simulink model "stage1_ddc"  (R2012b)
settings: Solver=FixedStepDiscrete  SolverMode=SingleTasking  StartTime=0.0  StopTime=T  RelTol=1e-3
undefined symbols (not defined in the file): cb0, cb1, cb2, cb3, cb4, cb5, cb6, cb7, dphi, Dphi, phi0
libraries: xbsIndex_r4 x332, unit_testing x23, filters x8, r2daq_blocks x5, synths x1, xps_library x1
(part 1 of 10)
settings Model: Creator=ayoung  LastModifiedBy=ayoung

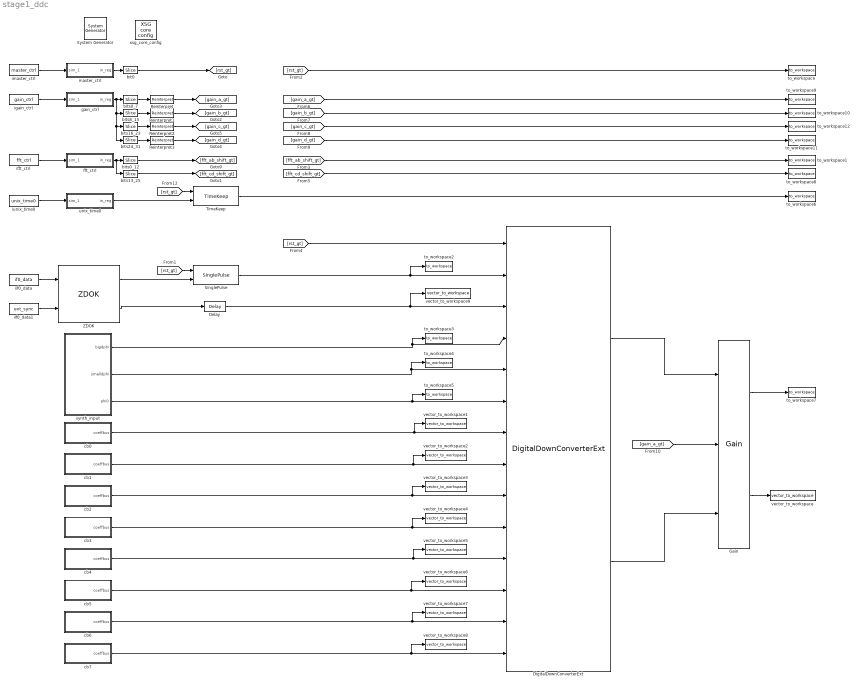
== system stage1_ddc ==
  " System Generator" : xbsIndex_r4/ System Generator  Tag=genX  xilinxfamily=Kintex7  part=xc7k325t  speed=-3  package=fbg676  synthesis_tool=XST  clock_wrapper=Clock Enables  directory=./netlist  proj_type=Project Navigator  Synth_file=XST Defaults  Impl_file=ISE Defaults  testbench=off  simulink_period=1  sysclk_period=10  dcm_input_clock_period=10  incr_netlist=off  trim_vbits=Everywhere in SubSystem  dbl_ovrd=According to Block Masks  core_generation=According to Block Masks  run_coregen=off  deprecated_control=off  eval_field=0  block_type=sysgen
  Delay : xbsIndex_r4/Delay  rst=off  infoeditControl=Selection of Reset will increase slice count due to use of real FFs and instead of SRLs  en=off  latency=1  dbl_ovrd=off  reg_retiming=off  block_type=delay
  DigitalDownConverterExt : r2daq_blocks/DigitalDownConverterExt
      link override bus_mul_cosine/a_debus: outputNum=1
      link override bus_mul_cosine/b_debus: outputNum=1
      link override bus_mul_sine/a_debus: outputNum=1
      link override bus_mul_sine/b_debus: outputNum=1
      link override ifir/bus_del1/din_expand: outputNum=1
      link override ifir/bus_del2/din_expand: outputNum=1
      link override ifir/bus_del3/din_expand: outputNum=1
      link override ifir/bus_del4/din_expand: outputNum=1
      link override ifir/bus_del5/din_expand: outputNum=1
      link override ifir/bus_del6/din_expand: outputNum=1
      link override ifir/bus_del7/din_expand: outputNum=1
      link override ifir/bus_mul0/a_debus: outputNum=1
      link override ifir/bus_mul0/b_debus: outputNum=1
      link override ifir/bus_mul1/a_debus: outputNum=1
      link override ifir/bus_mul1/b_debus: outputNum=1
      link override ifir/bus_mul2/a_debus: outputNum=1
      link override ifir/bus_mul2/b_debus: outputNum=1
      link override ifir/bus_mul3/a_debus: outputNum=1
      link override ifir/bus_mul3/b_debus: outputNum=1
      link override ifir/bus_mul4/a_debus: outputNum=1
      link override ifir/bus_mul4/b_debus: outputNum=1
      link override ifir/bus_mul5/a_debus: outputNum=1
      link override ifir/bus_mul5/b_debus: outputNum=1
      link override ifir/bus_mul6/a_debus: outputNum=1
      link override ifir/bus_mul6/b_debus: outputNum=1
      link override ifir/bus_mul7/a_debus: outputNum=1
      link override ifir/bus_mul7/b_debus: outputNum=1
      link override qfir/bus_del1/din_expand: outputNum=1
      link override qfir/bus_del2/din_expand: outputNum=1
      link override qfir/bus_del3/din_expand: outputNum=1
      link override qfir/bus_del4/din_expand: outputNum=1
      link override qfir/bus_del5/din_expand: outputNum=1
      link override qfir/bus_del6/din_expand: outputNum=1
      link override qfir/bus_del7/din_expand: outputNum=1
      link override qfir/bus_mul0/a_debus: outputNum=1
      link override qfir/bus_mul0/b_debus: outputNum=1
      link override qfir/bus_mul1/a_debus: outputNum=1
      link override qfir/bus_mul1/b_debus: outputNum=1
      link override qfir/bus_mul2/a_debus: outputNum=1
      link override qfir/bus_mul2/b_debus: outputNum=1
      link override qfir/bus_mul3/a_debus: outputNum=1
      link override qfir/bus_mul3/b_debus: outputNum=1
      link override qfir/bus_mul4/a_debus: outputNum=1
      link override qfir/bus_mul4/b_debus: outputNum=1
      link override qfir/bus_mul5/a_debus: outputNum=1
      link override qfir/bus_mul5/b_debus: outputNum=1
      link override qfir/bus_mul6/a_debus: outputNum=1
      link override qfir/bus_mul6/b_debus: outputNum=1
      link override qfir/bus_mul7/a_debus: outputNum=1
      link override qfir/bus_mul7/b_debus: outputNum=1
  Gain : r2daq_blocks/Gain
  Reinterpret{,1..3} (4 alike) : xbsIndex_r4/Reinterpret  force_arith_type=on  arith_type="Signed  (2's comp)"  force_bin_pt=on  bin_pt=4  block_type=reinterpret
  SinglePulse : r2daq_blocks/SinglePulse
  TimeKeep : r2daq_blocks/TimeKeep
  ZDOK : r2daq_blocks/ZDOK  zdok_slot=ZDOK 1  freq_nyq=1600
      link override asiaa_adc5g/a0: Port=1
      link override asiaa_adc5g/a1: Port=2
      link override asiaa_adc5g/a10: Port=11
      link override asiaa_adc5g/a11: Port=12
      link override asiaa_adc5g/a12: Port=13
      link override asiaa_adc5g/a13: Port=14
      link override asiaa_adc5g/a14: Port=15
      link override asiaa_adc5g/a15: Port=16
      link override asiaa_adc5g/a2: Port=3
      link override asiaa_adc5g/a3: Port=4
      link override asiaa_adc5g/a4: Port=5
      link override asiaa_adc5g/a5: Port=6
      link override asiaa_adc5g/a6: Port=7
      link override asiaa_adc5g/a7: Port=8
      link override asiaa_adc5g/a8: Port=9
      link override asiaa_adc5g/a9: Port=10
      link override asiaa_adc5g/bias_a: Bias=128
      link override asiaa_adc5g/delay_a0: DelayLength=2
      link override asiaa_adc5g/delay_a1: DelayLength=1
      link override asiaa_adc5g/delay_a10: DelayLength=1
      link override asiaa_adc5g/delay_a11: DelayLength=1
      link override asiaa_adc5g/delay_a12: DelayLength=1
      link override asiaa_adc5g/delay_a13: DelayLength=1
      link override asiaa_adc5g/delay_a14: DelayLength=1
      link override asiaa_adc5g/delay_a15: DelayLength=1
      link override asiaa_adc5g/delay_a2: DelayLength=1
      link override asiaa_adc5g/delay_a3: DelayLength=1
      link override asiaa_adc5g/delay_a4: DelayLength=1
      link override asiaa_adc5g/delay_a5: DelayLength=1
      link override asiaa_adc5g/delay_a6: DelayLength=1
      link override asiaa_adc5g/delay_a7: DelayLength=1
      link override asiaa_adc5g/delay_a8: DelayLength=1
      link override asiaa_adc5g/delay_a9: DelayLength=1
      link override asiaa_adc5g/downsample_a0: N=16  phase=0  RateOptions=Allow multirate processing  ic=0
      link override asiaa_adc5g/downsample_a1: N=16  phase=1  RateOptions=Allow multirate processing  ic=0
      link override asiaa_adc5g/downsample_a10: N=16  phase=10  RateOptions=Allow multirate processing  ic=0
      link override asiaa_adc5g/downsample_a11: N=16  phase=11  RateOptions=Allow multirate processing  ic=0
      link override asiaa_adc5g/downsample_a12: N=16  phase=12  RateOptions=Allow multirate processing  ic=0
      link override asiaa_adc5g/downsample_a13: N=16  phase=13  RateOptions=Allow multirate processing  ic=0
      link override asiaa_adc5g/downsample_a14: N=16  phase=14  RateOptions=Allow multirate processing  ic=0
      link override asiaa_adc5g/downsample_a15: N=16  phase=15  RateOptions=Allow multirate processing  ic=0
      link override asiaa_adc5g/downsample_a2: N=16  phase=2  RateOptions=Allow multirate processing  ic=0
      link override asiaa_adc5g/downsample_a3: N=16  phase=3  RateOptions=Allow multirate processing  ic=0
      link override asiaa_adc5g/downsample_a4: N=16  phase=4  RateOptions=Allow multirate processing  ic=0
      link override asiaa_adc5g/downsample_a5: N=16  phase=5  RateOptions=Allow multirate processing  ic=0
      link override asiaa_adc5g/downsample_a6: N=16  phase=6  RateOptions=Allow multirate processing  ic=0
      link override asiaa_adc5g/downsample_a7: N=16  phase=7  RateOptions=Allow multirate processing  ic=0
      link override asiaa_adc5g/downsample_a8: N=16  phase=8  RateOptions=Allow multirate processing  ic=0
      link override asiaa_adc5g/downsample_a9: N=16  phase=9  RateOptions=Allow multirate processing  ic=0
      link override asiaa_adc5g/gain_a: Gain=128
      link override asiaa_adc5g/sim_a: Port=1
      link override asiaa_adc5g/sim_sync: Port=2
      link override asiaa_adc5g/simulink_need_slupdate_PID_Controller_with_Approximate_Derivative_sync: arith_type=Boolean
      link override asiaa_adc5g/simulink_need_slupdate_PID_Controller_with_Approximate_Derivative_user_data_i0: arith_type=Unsigned  n_bits=8  bin_pt=0  quantization=Truncate  overflow=Wrap
      link override asiaa_adc5g/simulink_need_slupdate_PID_Controller_with_Approximate_Derivative_user_data_i1: arith_type=Unsigned  n_bits=8  bin_pt=0  quantization=Truncate  overflow=Wrap
      link override asiaa_adc5g/simulink_need_slupdate_PID_Controller_with_Approximate_Derivative_user_data_i2: arith_type=Unsigned  n_bits=8  bin_pt=0  quantization=Truncate  overflow=Wrap
      link override asiaa_adc5g/simulink_need_slupdate_PID_Controller_with_Approximate_Derivative_user_data_i3: arith_type=Unsigned  n_bits=8  bin_pt=0  quantization=Truncate  overflow=Wrap
      link override asiaa_adc5g/simulink_need_slupdate_PID_Controller_with_Approximate_Derivative_user_data_i4: arith_type=Unsigned  n_bits=8  bin_pt=0  quantization=Truncate  overflow=Wrap
      link override asiaa_adc5g/simulink_need_slupdate_PID_Controller_with_Approximate_Derivative_user_data_i5: arith_type=Unsigned  n_bits=8  bin_pt=0  quantization=Truncate  overflow=Wrap
      link override asiaa_adc5g/simulink_need_slupdate_PID_Controller_with_Approximate_Derivative_user_data_i6: arith_type=Unsigned  n_bits=8  bin_pt=0  quantization=Truncate  overflow=Wrap
      link override asiaa_adc5g/simulink_need_slupdate_PID_Controller_with_Approximate_Derivative_user_data_i7: arith_type=Unsigned  n_bits=8  bin_pt=0  quantization=Truncate  overflow=Wrap
      link override asiaa_adc5g/simulink_need_slupdate_PID_Controller_with_Approximate_Derivative_user_data_q0: arith_type=Unsigned  n_bits=8  bin_pt=0  quantization=Truncate  overflow=Wrap
      link override asiaa_adc5g/simulink_need_slupdate_PID_Controller_with_Approximate_Derivative_user_data_q1: arith_type=Unsigned  n_bits=8  bin_pt=0  quantization=Truncate  overflow=Wrap
      link override asiaa_adc5g/simulink_need_slupdate_PID_Controller_with_Approximate_Derivative_user_data_q2: arith_type=Unsigned  n_bits=8  bin_pt=0  quantization=Truncate  overflow=Wrap
      link override asiaa_adc5g/simulink_need_slupdate_PID_Controller_with_Approximate_Derivative_user_data_q3: arith_type=Unsigned  n_bits=8  bin_pt=0  quantization=Truncate  overflow=Wrap
      link override asiaa_adc5g/simulink_need_slupdate_PID_Controller_with_Approximate_Derivative_user_data_q4: arith_type=Unsigned  n_bits=8  bin_pt=0  quantization=Truncate  overflow=Wrap
      link override asiaa_adc5g/simulink_need_slupdate_PID_Controller_with_Approximate_Derivative_user_data_q5: arith_type=Unsigned  n_bits=8  bin_pt=0  quantization=Truncate  overflow=Wrap
      link override asiaa_adc5g/simulink_need_slupdate_PID_Controller_with_Approximate_Derivative_user_data_q6: arith_type=Unsigned  n_bits=8  bin_pt=0  quantization=Truncate  overflow=Wrap
      link override asiaa_adc5g/simulink_need_slupdate_PID_Controller_with_Approximate_Derivative_user_data_q7: arith_type=Unsigned  n_bits=8  bin_pt=0  quantization=Truncate  overflow=Wrap
      link override asiaa_adc5g/sync_out: Port=17
  bit0 : xbsIndex_r4/Slice  nbits=1  boolean_output=on  mode=Lower Bit Location + Width  bit1=0  base1=LSB of Input  bit0=0  base0=LSB of Input  dbl_ovrd=off  block_type=slice
  bits0_12 : xbsIndex_r4/Slice  nbits=13  boolean_output=off  mode=Lower Bit Location + Width  bit1=0  base1=LSB of Input  bit0=0  base0=LSB of Input  dbl_ovrd=off  block_type=slice
  bits0_7 : xbsIndex_r4/Slice  nbits=8  boolean_output=off  mode=Lower Bit Location + Width  bit1=0  base1=LSB of Input  bit0=0  base0=LSB of Input  dbl_ovrd=off  block_type=slice
  bits13_25 : xbsIndex_r4/Slice  nbits=13  boolean_output=off  mode=Lower Bit Location + Width  bit1=0  base1=LSB of Input  bit0=13  base0=LSB of Input  dbl_ovrd=off  block_type=slice
  bits16_23 : xbsIndex_r4/Slice  nbits=8  boolean_output=off  mode=Lower Bit Location + Width  bit1=0  base1=LSB of Input  bit0=8  base0=LSB of Input  dbl_ovrd=off  block_type=slice
  bits24_31 : xbsIndex_r4/Slice  nbits=8  boolean_output=off  mode=Lower Bit Location + Width  bit1=0  base1=LSB of Input  bit0=8  base0=LSB of Input  dbl_ovrd=off  block_type=slice
  bits8_15 : xbsIndex_r4/Slice  nbits=8  boolean_output=off  mode=Lower Bit Location + Width  bit1=0  base1=LSB of Input  bit0=8  base0=LSB of Input  dbl_ovrd=off  block_type=slice
  cb0 : Subsystem  AncestorBlock=filters/coeff_16x8bit_bus  mask(coeff_16x8bit_bus){io_delay=3, sim_in=on, coeff=cb0}
      mask prompts: io_delay "I/O delay for registers"; sim_in "Provide sim input?"; coeff "Coefficients (4 x uint32)"
      mask help:
      | Provides 16x8bit coefficients on a single bus.
      |
      | The coefficients are set in 4x32bit software registers.
      |
      | The I/O delay of the internal registers can be set, as well as an optional simulation input to each.
      mask init:
      | %for ii=0:3
      | %    swr = [gcb sprintf('/g%d',ii)];
      | %    set_param(swr,'sim_port',sim_in);
      | %    set_param(swr,'io_delay',num2str(io_delay));
      | %end
      | coeff_16x8bit_bus_init(gcb,...
      |     'io_delay',io_delay,...
      |     'sim_in',sim_in,...
      |     'coeff',coeff);
      mask Callback sim_in:
      | if strcmpi(get_param(gcb,'sim_in'),'off')
      |     set_param(gcb,'MaskEnables',{'on';'on';'off'});
      | else
      |     set_param(gcb,'MaskEnables',{'on';'on';'on'});
      | end
  cb1 : Subsystem  AncestorBlock=filters/coeff_16x8bit_bus  mask(coeff_16x8bit_bus){io_delay=3, sim_in=on, coeff=cb1}
      mask prompts: io_delay "I/O delay for registers"; sim_in "Provide sim input?"; coeff "Coefficients (4 x uint32)"
      mask help:
      | Provides 16x8bit coefficients on a single bus.
      |
      | The coefficients are set in 4x32bit software registers.
      |
      | The I/O delay of the internal registers can be set, as well as an optional simulation input to each.
      mask init: same as stage1_ddc/cb0
      mask Callback sim_in:
      | if strcmpi(get_param(gcb,'sim_in'),'off')
      |     set_param(gcb,'MaskEnables',{'on';'on';'off'});
      | else
      |     set_param(gcb,'MaskEnables',{'on';'on';'on'});
      | end
  cb2 : Subsystem  AncestorBlock=filters/coeff_16x8bit_bus  mask(coeff_16x8bit_bus){io_delay=3, sim_in=on, coeff=cb2}
      mask prompts: io_delay "I/O delay for registers"; sim_in "Provide sim input?"; coeff "Coefficients (4 x uint32)"
      mask help:
      | Provides 16x8bit coefficients on a single bus.
      |
      | The coefficients are set in 4x32bit software registers.
      |
      | The I/O delay of the internal registers can be set, as well as an optional simulation input to each.
      mask init: same as stage1_ddc/cb0
      mask Callback sim_in:
      | if strcmpi(get_param(gcb,'sim_in'),'off')
      |     set_param(gcb,'MaskEnables',{'on';'on';'off'});
      | else
      |     set_param(gcb,'MaskEnables',{'on';'on';'on'});
      | end
  cb3 : Subsystem  AncestorBlock=filters/coeff_16x8bit_bus  mask(coeff_16x8bit_bus){io_delay=3, sim_in=on, coeff=cb3}
      mask prompts: io_delay "I/O delay for registers"; sim_in "Provide sim input?"; coeff "Coefficients (4 x uint32)"
      mask help:
      | Provides 16x8bit coefficients on a single bus.
      |
      | The coefficients are set in 4x32bit software registers.
      |
      | The I/O delay of the internal registers can be set, as well as an optional simulation input to each.
      mask init: same as stage1_ddc/cb0
      mask Callback sim_in:
      | if strcmpi(get_param(gcb,'sim_in'),'off')
      |     set_param(gcb,'MaskEnables',{'on';'on';'off'});
      | else
      |     set_param(gcb,'MaskEnables',{'on';'on';'on'});
      | end
  cb4 : Subsystem  AncestorBlock=filters/coeff_16x8bit_bus  mask(coeff_16x8bit_bus){io_delay=3, sim_in=on, coeff=cb4}
      mask prompts: io_delay "I/O delay for registers"; sim_in "Provide sim input?"; coeff "Coefficients (4 x uint32)"
      mask help:
      | Provides 16x8bit coefficients on a single bus.
      |
      | The coefficients are set in 4x32bit software registers.
      |
      | The I/O delay of the internal registers can be set, as well as an optional simulation input to each.
      mask init: same as stage1_ddc/cb0
      mask Callback sim_in:
      | if strcmpi(get_param(gcb,'sim_in'),'off')
      |     set_param(gcb,'MaskEnables',{'on';'on';'off'});
      | else
      |     set_param(gcb,'MaskEnables',{'on';'on';'on'});
      | end
  cb5 : Subsystem  AncestorBlock=filters/coeff_16x8bit_bus  mask(coeff_16x8bit_bus){io_delay=3, sim_in=on, coeff=cb5}
      mask prompts: io_delay "I/O delay for registers"; sim_in "Provide sim input?"; coeff "Coefficients (4 x uint32)"
      mask help:
      | Provides 16x8bit coefficients on a single bus.
      |
      | The coefficients are set in 4x32bit software registers.
      |
      | The I/O delay of the internal registers can be set, as well as an optional simulation input to each.
      mask init: same as stage1_ddc/cb0
      mask Callback sim_in:
      | if strcmpi(get_param(gcb,'sim_in'),'off')
      |     set_param(gcb,'MaskEnables',{'on';'on';'off'});
      | else
      |     set_param(gcb,'MaskEnables',{'on';'on';'on'});
      | end
  cb6 : Subsystem  AncestorBlock=filters/coeff_16x8bit_bus  mask(coeff_16x8bit_bus){io_delay=3, sim_in=on, coeff=cb6}
      mask prompts: io_delay "I/O delay for registers"; sim_in "Provide sim input?"; coeff "Coefficients (4 x uint32)"
      mask help:
      | Provides 16x8bit coefficients on a single bus.
      |
      | The coefficients are set in 4x32bit software registers.
      |
      | The I/O delay of the internal registers can be set, as well as an optional simulation input to each.
      mask init: same as stage1_ddc/cb0
      mask Callback sim_in:
      | if strcmpi(get_param(gcb,'sim_in'),'off')
      |     set_param(gcb,'MaskEnables',{'on';'on';'off'});
      | else
      |     set_param(gcb,'MaskEnables',{'on';'on';'on'});
      | end
  cb7 : Subsystem  AncestorBlock=filters/coeff_16x8bit_bus  mask(coeff_16x8bit_bus){io_delay=3, sim_in=on, coeff=cb7}
      mask prompts: io_delay "I/O delay for registers"; sim_in "Provide sim input?"; coeff "Coefficients (4 x uint32)"
      mask help:
      | Provides 16x8bit coefficients on a single bus.
      |
      | The coefficients are set in 4x32bit software registers.
      |
      | The I/O delay of the internal registers can be set, as well as an optional simulation input to each.
      mask init: same as stage1_ddc/cb0
      mask Callback sim_in:
      | if strcmpi(get_param(gcb,'sim_in'),'off')
      |     set_param(gcb,'MaskEnables',{'on';'on';'off'});
      | else
      |     set_param(gcb,'MaskEnables',{'on';'on';'on'});
      | end
  fft_ctrl : Subsystem  Tag=xps:sw_reg  AncestorBlock=xps_library/software_register  mask(swreg){mode=one value, io_dir=From Processor, io_delay=0, sample_period=1, names=reg, bitwidths=32, arith_types=0, bin_pts=0, sim_port=on, show_format=off}
      mask prompts: io_dir "I/O direction"; io_delay "I/O delay"; sample_period "Sample period"; names "Name:"; bitwidths "Bitwidth:"; arith_types "Type (ufix=0, fix=1, bool=2):"; bin_pts "Binary pt:"; sim_port "Provide sim input/output?"; show_format "Print format string?"
      mask init:
      | swreg_init(gcb)
      settings: AttributesFormatString=1input
      mask TypeOptions mode: one value | fields of equal size | fields of arbitrary size
      mask Callback mode: swreg_cb(gcb);
      mask TypeOptions io_dir: To Processor | From Processor
      mask Callback io_dir:
      | mask_enables = get_param(gcb, 'MaskEnables');
      | mask_names = get_param(gcb, 'MaskNames');
      | if strcmp(get_param(gcb, 'io_dir'), 'To Processor'),
      |     mask_enables{ismember(mask_names, 'sample_period')} = 'off';
      | else
      |     mask_enables{ismember(mask_names, 'sample_period')} = 'on';
      | end
      | set_param(gcb, 'MaskEnables', mask_enables);
      mask Callback bitwidths:
      | swreg_maskcheck(gcb);
      | % blk = gcb;
      | % mode = get_param(blk, 'mode');
      | % current_widths = eval(get_param(blk, 'bitwidths'));
      | % if (strcmp(mode, 'one value') || strcmp(mode, 'fields of equal size')) && (length(current_widths) > 1),
      | %     error('Only one width may be specified for this mode.');
      | % elseif strcmp(mode, 'fields of arbitrary size')
      | %     current_names = textscan(strtrim(strrep(strrep(get_param(blk, 'names'), ']', ''), '[', '')), '%s');
      | %     current_names = current_names{1};
      | %     numios = length(current_names);
      | %     if length(current_widths) ~= numios,
      | %         error('%d field names specified, but %d widths?', numios, length(current_widths));
      | %     end
      | % end
      | % total_width = 0;
      | % for ctr = 1 : length(current_widths),
      | %     total_width = total_width + current_widths(ctr);
      | % end
      | % if total_width > 32,
      | %     error('Total width must be 32 or less, set to %d.', total_width);
      | % end
      mask Callback arith_types:
      | [numios, ~, ~, ~, current_types] = swreg_maskcheck(gcb);
      | % blk = gcb;
      | % mode = get_param(blk, 'mode');
      | % current_types = eval(get_param(blk, 'arith_types'));
      | % numios = length(current_types);
      | % if (strcmp(mode, 'one value') || strcmp(mode, 'fields of equal size')) && (length(current_types) > 1),
      | %     error('Only one type may be specified for this mode.');
      | % elseif strcmp(mode, 'fields of arbitrary size')
      | %     current_names = textscan(strtrim(strrep(strrep(get_param(blk, 'names'), ']', ''), '[', '')), '%s');
      | %     current_names = current_names{1};
      | %     numios = length(current_names);
      | %     if length(current_types) ~= numios,
      | %         error('%d field names specified, but %d types?', numios, length(current_types));
      | %     end
      | % end
      | problem = 0;
      | for ctr = 1 : numios,
      |     t = current_types(ctr);
      |     if (t < 0) || (t > 2),
      |         problem = t;
      |         ctr = numios + 1;
      |     end
      | end
      | if problem ~= 0,
      |     error('Type cannot be %i, must be 0, 1 or 2.', problem);
      | end
      mask Callback bin_pts:
      | swreg_maskcheck(gcb);
      | % blk = gcb;
      | % mode = get_param(blk, 'mode');
      | % current_bins = eval(get_param(blk, 'bin_pts'));
      | % if (strcmp(mode, 'one value') || strcmp(mode, 'fields of equal size')) && (length(current_bins) > 1),
      | %     error('Only one binary pt may be specified for this mode.');
      | % elseif strcmp(mode, 'fields of arbitrary size')
      | %     current_names = textscan(strtrim(strrep(strrep(get_param(blk, 'names'), ']', ''), '[', '')), '%s');
      | %     current_names = current_names{1};
      | %     numios = length(current_names);
      | %     if length(current_bins) ~= numios,
      | %         error('%d field names specified, but %d binary pts?', numios, length(current_bins));
      | %     end
      | % end
  gain_ctrl : Subsystem  Tag=xps:sw_reg  AncestorBlock=xps_library/software_register  mask(swreg){mode=one value, io_dir=From Processor, io_delay=0, sample_period=1, names=reg, bitwidths=32, arith_types=0, bin_pts=0, sim_port=on, show_format=off}
      mask prompts: io_dir "I/O direction"; io_delay "I/O delay"; sample_period "Sample period"; names "Name:"; bitwidths "Bitwidth:"; arith_types "Type (ufix=0, fix=1, bool=2):"; bin_pts "Binary pt:"; sim_port "Provide sim input/output?"; show_format "Print format string?"
      mask init:
      | swreg_init(gcb)
      settings: AttributesFormatString=1input
      mask TypeOptions mode: one value | fields of equal size | fields of arbitrary size
      mask Callback mode: swreg_cb(gcb);
      mask TypeOptions io_dir: To Processor | From Processor
      mask Callback io_dir:
      | mask_enables = get_param(gcb, 'MaskEnables');
      | mask_names = get_param(gcb, 'MaskNames');
      | if strcmp(get_param(gcb, 'io_dir'), 'To Processor'),
      |     mask_enables{ismember(mask_names, 'sample_period')} = 'off';
      | else
      |     mask_enables{ismember(mask_names, 'sample_period')} = 'on';
      | end
      | set_param(gcb, 'MaskEnables', mask_enables);
      mask Callback bitwidths:
      | swreg_maskcheck(gcb);
      | % blk = gcb;
      | % mode = get_param(blk, 'mode');
      | % current_widths = eval(get_param(blk, 'bitwidths'));
      | % if (strcmp(mode, 'one value') || strcmp(mode, 'fields of equal size')) && (length(current_widths) > 1),
      | %     error('Only one width may be specified for this mode.');
      | % elseif strcmp(mode, 'fields of arbitrary size')
      | %     current_names = textscan(strtrim(strrep(strrep(get_param(blk, 'names'), ']', ''), '[', '')), '%s');
      | %     current_names = current_names{1};
      | %     numios = length(current_names);
      | %     if length(current_widths) ~= numios,
      | %         error('%d field names specified, but %d widths?', numios, length(current_widths));
      | %     end
      | % end
      | % total_width = 0;
      | % for ctr = 1 : length(current_widths),
      | %     total_width = total_width + current_widths(ctr);
      | % end
      | % if total_width > 32,
      | %     error('Total width must be 32 or less, set to %d.', total_width);
      | % end
      mask Callback arith_types:
      | [numios, ~, ~, ~, current_types] = swreg_maskcheck(gcb);
      | % blk = gcb;
      | % mode = get_param(blk, 'mode');
      | % current_types = eval(get_param(blk, 'arith_types'));
      | % numios = length(current_types);
      | % if (strcmp(mode, 'one value') || strcmp(mode, 'fields of equal size')) && (length(current_types) > 1),
      | %     error('Only one type may be specified for this mode.');
      | % elseif strcmp(mode, 'fields of arbitrary size')
      | %     current_names = textscan(strtrim(strrep(strrep(get_param(blk, 'names'), ']', ''), '[', '')), '%s');
      | %     current_names = current_names{1};
      | %     numios = length(current_names);
      | %     if length(current_types) ~= numios,
      | %         error('%d field names specified, but %d types?', numios, length(current_types));
      | %     end
      | % end
      | problem = 0;
      | for ctr = 1 : numios,
      |     t = current_types(ctr);
      |     if (t < 0) || (t > 2),
      |         problem = t;
      |         ctr = numios + 1;
      |     end
      | end
      | if problem ~= 0,
      |     error('Type cannot be %i, must be 0, 1 or 2.', problem);
      | end
      mask Callback bin_pts:
      | swreg_maskcheck(gcb);
      | % blk = gcb;
      | % mode = get_param(blk, 'mode');
      | % current_bins = eval(get_param(blk, 'bin_pts'));
      | % if (strcmp(mode, 'one value') || strcmp(mode, 'fields of equal size')) && (length(current_bins) > 1),
      | %     error('Only one binary pt may be specified for this mode.');
      | % elseif strcmp(mode, 'fields of arbitrary size')
      | %     current_names = textscan(strtrim(strrep(strrep(get_param(blk, 'names'), ']', ''), '[', '')), '%s');
      | %     current_names = current_names{1};
      | %     numios = length(current_names);
      | %     if length(current_bins) ~= numios,
      | %         error('%d field names specified, but %d binary pts?', numios, length(current_bins));
      | %     end
      | % end
  ifft_ctrl : FromWorkspace  VariableName=fft_ctrl  SampleTime=1/16  Interpolate=off  OutputAfterFinalValue=Holding final value
  igain_ctrl : FromWorkspace  VariableName=gain_ctrl  SampleTime=1/16  Interpolate=off  OutputAfterFinalValue=Holding final value
  iif0_data : FromWorkspace  VariableName=if0_data  SampleTime=1/16  Interpolate=off  OutputAfterFinalValue=Holding final value
  iif0_data1 : FromWorkspace  VariableName=ext_sync  SampleTime=1/16  Interpolate=off  OutputAfterFinalValue=Holding final value
  imaster_ctrl : FromWorkspace  VariableName=master_ctrl  SampleTime=1/16  Interpolate=off  OutputAfterFinalValue=Holding final value
  iunix_time0 : FromWorkspace  VariableName=unix_time0  SampleTime=1/16  Interpolate=off  OutputAfterFinalValue=Holding final value
  master_ctrl : Subsystem  Tag=xps:sw_reg  AncestorBlock=xps_library/software_register  mask(swreg){mode=one value, io_dir=From Processor, io_delay=0, sample_period=1, names=reg, bitwidths=32, arith_types=0, bin_pts=0, sim_port=on, show_format=off}
      mask prompts: io_dir "I/O direction"; io_delay "I/O delay"; sample_period "Sample period"; names "Name:"; bitwidths "Bitwidth:"; arith_types "Type (ufix=0, fix=1, bool=2):"; bin_pts "Binary pt:"; sim_port "Provide sim input/output?"; show_format "Print format string?"
      mask init:
      | swreg_init(gcb)
      settings: AttributesFormatString=1input
      mask TypeOptions mode: one value | fields of equal size | fields of arbitrary size
      mask Callback mode: swreg_cb(gcb);
      mask TypeOptions io_dir: To Processor | From Processor
      mask Callback io_dir:
      | mask_enables = get_param(gcb, 'MaskEnables');
      | mask_names = get_param(gcb, 'MaskNames');
      | if strcmp(get_param(gcb, 'io_dir'), 'To Processor'),
      |     mask_enables{ismember(mask_names, 'sample_period')} = 'off';
      | else
      |     mask_enables{ismember(mask_names, 'sample_period')} = 'on';
      | end
      | set_param(gcb, 'MaskEnables', mask_enables);
      mask Callback bitwidths:
      | swreg_maskcheck(gcb);
      | % blk = gcb;
      | % mode = get_param(blk, 'mode');
      | % current_widths = eval(get_param(blk, 'bitwidths'));
      | % if (strcmp(mode, 'one value') || strcmp(mode, 'fields of equal size')) && (length(current_widths) > 1),
      | %     error('Only one width may be specified for this mode.');
      | % elseif strcmp(mode, 'fields of arbitrary size')
      | %     current_names = textscan(strtrim(strrep(strrep(get_param(blk, 'names'), ']', ''), '[', '')), '%s');
      | %     current_names = current_names{1};
      | %     numios = length(current_names);
      | %     if length(current_widths) ~= numios,
      | %         error('%d field names specified, but %d widths?', numios, length(current_widths));
      | %     end
      | % end
      | % total_width = 0;
      | % for ctr = 1 : length(current_widths),
      | %     total_width = total_width + current_widths(ctr);
      | % end
      | % if total_width > 32,
      | %     error('Total width must be 32 or less, set to %d.', total_width);
      | % end
      mask Callback arith_types:
      | [numios, ~, ~, ~, current_types] = swreg_maskcheck(gcb);
      | % blk = gcb;
      | % mode = get_param(blk, 'mode');
      | % current_types = eval(get_param(blk, 'arith_types'));
      | % numios = length(current_types);
      | % if (strcmp(mode, 'one value') || strcmp(mode, 'fields of equal size')) && (length(current_types) > 1),
      | %     error('Only one type may be specified for this mode.');
      | % elseif strcmp(mode, 'fields of arbitrary size')
      | %     current_names = textscan(strtrim(strrep(strrep(get_param(blk, 'names'), ']', ''), '[', '')), '%s');
      | %     current_names = current_names{1};
      | %     numios = length(current_names);
      | %     if length(current_types) ~= numios,
      | %         error('%d field names specified, but %d types?', numios, length(current_types));
      | %     end
      | % end
      | problem = 0;
      | for ctr = 1 : numios,
      |     t = current_types(ctr);
      |     if (t < 0) || (t > 2),
      |         problem = t;
      |         ctr = numios + 1;
      |     end
      | end
      | if problem ~= 0,
      |     error('Type cannot be %i, must be 0, 1 or 2.', problem);
      | end
      mask Callback bin_pts:
      | swreg_maskcheck(gcb);
      | % blk = gcb;
      | % mode = get_param(blk, 'mode');
      | % current_bins = eval(get_param(blk, 'bin_pts'));
      | % if (strcmp(mode, 'one value') || strcmp(mode, 'fields of equal size')) && (length(current_bins) > 1),
      | %     error('Only one binary pt may be specified for this mode.');
      | % elseif strcmp(mode, 'fields of arbitrary size')
      | %     current_names = textscan(strtrim(strrep(strrep(get_param(blk, 'names'), ']', ''), '[', '')), '%s');
      | %     current_names = current_names{1};
      | %     numios = length(current_names);
      | %     if length(current_bins) ~= numios,
      | %         error('%d field names specified, but %d binary pts?', numios, length(current_bins));
      | %     end
      | % end
  synth_input : Subsystem  AncestorBlock=synths/synth_input  mask(synth_input){io_delay=3, sim_in=on, dphi=dphi, demux_dphi=Dphi, phi0=phi0}
      mask prompts: io_delay "I/O delay"; sim_in "Sim input?"; dphi "Phase increment per sample"; demux_dphi "Phase increment per demux set"; phi0 "Phase offset"
      mask help:
      | Defines input for synth using a single 32bit software register.
      |
      | I/O delay and optional simulated input for the register are configurable.
      |
      | If simulated input is set, a feed is internally generated using the given parameters for phase increment and offset.
      mask init:
      | synth_input_init(gcb,...
      |     'io_delay',io_delay,...
      |     'sim_in',sim_in,...
      |     'dphi',dphi,...
      |     'demux_dphi',demux_dphi,...
      |     'phi0',phi0);
      mask Callback sim_in:
      | if strcmpi(get_param(gcb,'sim_in'),'on')
      |     set_param(gcb,'MaskEnables',{'on';'on';'on';'on';'on'});
      | else
      |     set_param(gcb,'MaskEnables',{'on';'on';'off';'off';'off'});
      | end
  to_workspace : unit_testing/to_workspace  var_name=rst
  to_workspace1 : unit_testing/to_workspace  var_name=fft_ab_shift
  to_workspace10 : unit_testing/to_workspace  var_name=gain_b
  to_workspace11 : unit_testing/to_workspace  var_name=gain_d
  to_workspace12 : unit_testing/to_workspace  var_name=gain_c
  to_workspace2 : unit_testing/to_workspace  var_name=sync_in
  to_workspace3 : unit_testing/to_workspace  var_name=Ddphi
  to_workspace4 : unit_testing/to_workspace  var_name=dphi
  to_workspace5 : unit_testing/to_workspace  var_name=phi0
  to_workspace6 : unit_testing/to_workspace  var_name=ut
  to_workspace7 : unit_testing/to_workspace  var_name=sync_out
  to_workspace8 : unit_testing/to_workspace  var_name=fft_cd_shift
  to_workspace9 : unit_testing/to_workspace  var_name=gain_a
  unix_time0 : Subsystem  Tag=xps:sw_reg  AncestorBlock=xps_library/software_register  mask(swreg){mode=one value, io_dir=From Processor, io_delay=0, sample_period=1, names=reg, bitwidths=32, arith_types=0, bin_pts=0, sim_port=on, show_format=off}
      mask prompts: io_dir "I/O direction"; io_delay "I/O delay"; sample_period "Sample period"; names "Name:"; bitwidths "Bitwidth:"; arith_types "Type (ufix=0, fix=1, bool=2):"; bin_pts "Binary pt:"; sim_port "Provide sim input/output?"; show_format "Print format string?"
      mask init:
      | swreg_init(gcb)
      settings: AttributesFormatString=1input
      mask TypeOptions mode: one value | fields of equal size | fields of arbitrary size
      mask Callback mode: swreg_cb(gcb);
      mask TypeOptions io_dir: To Processor | From Processor
      mask Callback io_dir:
      | mask_enables = get_param(gcb, 'MaskEnables');
      | mask_names = get_param(gcb, 'MaskNames');
      | if strcmp(get_param(gcb, 'io_dir'), 'To Processor'),
      |     mask_enables{ismember(mask_names, 'sample_period')} = 'off';
      | else
      |     mask_enables{ismember(mask_names, 'sample_period')} = 'on';
      | end
      | set_param(gcb, 'MaskEnables', mask_enables);
      mask Callback bitwidths:
      | swreg_maskcheck(gcb);
      | % blk = gcb;
      | % mode = get_param(blk, 'mode');
      | % current_widths = eval(get_param(blk, 'bitwidths'));
      | % if (strcmp(mode, 'one value') || strcmp(mode, 'fields of equal size')) && (length(current_widths) > 1),
      | %     error('Only one width may be specified for this mode.');
      | % elseif strcmp(mode, 'fields of arbitrary size')
      | %     current_names = textscan(strtrim(strrep(strrep(get_param(blk, 'names'), ']', ''), '[', '')), '%s');
      | %     current_names = current_names{1};
      | %     numios = length(current_names);
      | %     if length(current_widths) ~= numios,
      | %         error('%d field names specified, but %d widths?', numios, length(current_widths));
      | %     end
      | % end
      | % total_width = 0;
      | % for ctr = 1 : length(current_widths),
      | %     total_width = total_width + current_widths(ctr);
      | % end
      | % if total_width > 32,
      | %     error('Total width must be 32 or less, set to %d.', total_width);
      | % end
      mask Callback arith_types:
      | [numios, ~, ~, ~, current_types] = swreg_maskcheck(gcb);
      | % blk = gcb;
      | % mode = get_param(blk, 'mode');
      | % current_types = eval(get_param(blk, 'arith_types'));
      | % numios = length(current_types);
      | % if (strcmp(mode, 'one value') || strcmp(mode, 'fields of equal size')) && (length(current_types) > 1),
      | %     error('Only one type may be specified for this mode.');
      | % elseif strcmp(mode, 'fields of arbitrary size')
      | %     current_names = textscan(strtrim(strrep(strrep(get_param(blk, 'names'), ']', ''), '[', '')), '%s');
      | %     current_names = current_names{1};
      | %     numios = length(current_names);
      | %     if length(current_types) ~= numios,
      | %         error('%d field names specified, but %d types?', numios, length(current_types));
      | %     end
      | % end
      | problem = 0;
      | for ctr = 1 : numios,
      |     t = current_types(ctr);
      |     if (t < 0) || (t > 2),
      |         problem = t;
      |         ctr = numios + 1;
      |     end
      | end
      | if problem ~= 0,
      |     error('Type cannot be %i, must be 0, 1 or 2.', problem);
      | end
      mask Callback bin_pts:
      | swreg_maskcheck(gcb);
      | % blk = gcb;
      | % mode = get_param(blk, 'mode');
      | % current_bins = eval(get_param(blk, 'bin_pts'));
      | % if (strcmp(mode, 'one value') || strcmp(mode, 'fields of equal size')) && (length(current_bins) > 1),
      | %     error('Only one binary pt may be specified for this mode.');
      | % elseif strcmp(mode, 'fields of arbitrary size')
      | %     current_names = textscan(strtrim(strrep(strrep(get_param(blk, 'names'), ']', ''), '[', '')), '%s');
      | %     current_names = current_names{1};
      | %     numios = length(current_names);
      | %     if length(current_bins) ~= numios,
      | %         error('%d field names specified, but %d binary pts?', numios, length(current_bins));
      | %     end
      | % end
  vector_to_workspace : unit_testing/vector_to_workspace  n_out=2  n_bits=25  bin_pt=16  arith_type=1  var_pfx=dout_c
      link override bus_expand/slice2: nbits=25  boolean_output=off  bit1=0
  vector_to_workspace1 : unit_testing/vector_to_workspace  n_out=16  n_bits=8  bin_pt=7  arith_type=1  var_pfx=cb0
  vector_to_workspace2 : unit_testing/vector_to_workspace  n_out=16  n_bits=8  bin_pt=7  arith_type=1  var_pfx=cb1
  vector_to_workspace3 : unit_testing/vector_to_workspace  n_out=16  n_bits=8  bin_pt=7  arith_type=1  var_pfx=cb2
  vector_to_workspace4 : unit_testing/vector_to_workspace  n_out=16  n_bits=8  bin_pt=7  arith_type=1  var_pfx=cb3
  vector_to_workspace5 : unit_testing/vector_to_workspace  n_out=16  n_bits=8  bin_pt=7  arith_type=1  var_pfx=cb4
  vector_to_workspace6 : unit_testing/vector_to_workspace  n_out=16  n_bits=8  bin_pt=7  arith_type=1  var_pfx=cb5
  vector_to_workspace7 : unit_testing/vector_to_workspace  n_out=16  n_bits=8  bin_pt=7  arith_type=1  var_pfx=cb6
  vector_to_workspace8 : unit_testing/vector_to_workspace  n_out=16  n_bits=8  bin_pt=7  arith_type=1  var_pfx=cb7
  vector_to_workspace9 : unit_testing/vector_to_workspace  n_out=16  n_bits=8  bin_pt=7  arith_type=1  var_pfx=din
  xsg_core_config : xps_library/XSG core config  Tag=xps:xsg  hw_sys=ROACH2:sx475t  clk_src=adc0_clk  ROACH_clk_src=sys_clk  ROACH2_clk_src=adc0_clk  MKDIG_clk_src=sys_clk  clk_rate=200  sample_period=1  synthesis_tool=XST
  wires:
  ZDOK/2 -> Delay/1
  iif0_data/1 -> ZDOK/1
  iif0_data1/1 -> ZDOK/2
  imaster_ctrl/1 -> master_ctrl/1(sim_1)
  master_ctrl/1(in_reg) -> bit0/1
  bit0/1 -> [rst_gt]
  iunix_time0/1 -> unix_time0/1(sim_1)
  ifft_ctrl/1 -> fft_ctrl/1(sim_1)
  unix_time0/1(in_reg) -> TimeKeep/2
  fft_ctrl/1(in_reg) -> bits13_25/1, bits0_12/1
  bits0_12/1 -> [fft_ab_shift_gt]
  [rst_gt] -> TimeKeep/1
  [rst_gt] -> SinglePulse/1
  [rst_gt] -> to_workspace/1
  [fft_ab_shift_gt] -> to_workspace1/1
  SinglePulse/1 -> to_workspace2/1, DigitalDownConverterExt/2
  Delay/1 -> vector_to_workspace9/1, DigitalDownConverterExt/3
  TimeKeep/1 -> to_workspace6/1
  ZDOK/1 -> SinglePulse/2
  [rst_gt] -> DigitalDownConverterExt/1
  synth_input/2(smalldphi) -> to_workspace4/1, DigitalDownConverterExt/5
  synth_input/1(bigdphi) -> to_workspace3/1, DigitalDownConverterExt/4
  synth_input/3(phi0) -> to_workspace5/1, DigitalDownConverterExt/6
  cb2/1(coeffbus) -> vector_to_workspace3/1, DigitalDownConverterExt/9
  cb6/1(coeffbus) -> vector_to_workspace7/1, DigitalDownConverterExt/13
  cb0/1(coeffbus) -> vector_to_workspace1/1, DigitalDownConverterExt/7
  cb1/1(coeffbus) -> vector_to_workspace2/1, DigitalDownConverterExt/8
  cb4/1(coeffbus) -> vector_to_workspace5/1, DigitalDownConverterExt/11
  cb5/1(coeffbus) -> vector_to_workspace6/1, DigitalDownConverterExt/12
  cb7/1(coeffbus) -> vector_to_workspace8/1, DigitalDownConverterExt/14
  cb3/1(coeffbus) -> vector_to_workspace4/1, DigitalDownConverterExt/10
  igain_ctrl/1 -> gain_ctrl/1(sim_1)
  bits13_25/1 -> [fft_cd_shift_gt]
  [fft_cd_shift_gt] -> to_workspace8/1
  gain_ctrl/1(in_reg) -> bits8_15/1, bits24_31/1, bits16_23/1, bits0_7/1
  bits0_7/1 -> Reinterpret/1
  bits8_15/1 -> Reinterpret1/1
  Reinterpret/1 -> [gain_a_gt]
  [gain_a_gt] -> to_workspace9/1
  Reinterpret1/1 -> [gain_b_gt]
  [gain_b_gt] -> to_workspace10/1
  bits16_23/1 -> Reinterpret2/1
  bits24_31/1 -> Reinterpret3/1
  Reinterpret2/1 -> [gain_c_gt]
  [gain_c_gt] -> to_workspace12/1
  Reinterpret3/1 -> [gain_d_gt]
  [gain_d_gt] -> to_workspace11/1
  DigitalDownConverterExt/2 -> Gain/3
  [gain_a_gt] -> Gain/2
  DigitalDownConverterExt/1 -> Gain/1
  Gain/1 -> to_workspace7/1
  Gain/2 -> vector_to_workspace/1
